simulink library "TB6612FNG"  (R2023b)
settings: Solver=VariableStepAuto  StartTime=0.0  StopTime=10.0  RelTol=1e-3
libraries: arduinolib x5
settings Model: Creator=user  LastModifiedBy=user

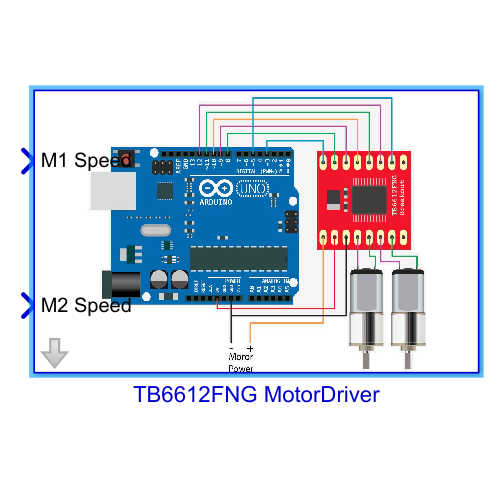
[thumbnail: Simulink's stored preview of the top-level diagram]
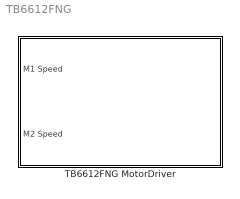
== system TB6612FNG ==
  TB6612FNG MotorDriver : Subsystem  mask{SetBYPin=8, InputAPin=7, EnablePin1=5, InputBPin=12, EnablePin2=6}
      mask TypeOptions SetBYPin: Digital Output2/pinNumber
      mask TypeOptions InputAPin: Digital Output/pinNumber
      mask TypeOptions EnablePin1: PWMSelection/pinNumber
      mask TypeOptions InputBPin: Digital Output1/pinNumber
      mask TypeOptions EnablePin2: PWMSelection1/pinNumber
      mask DialogControl DescGroupVar Prompt: TB6612FNG
      mask DialogControl DescTextVar Prompt: arduino：TB6612FNG Motor Driver
      mask Display: image('TB6612FNG.jpg');

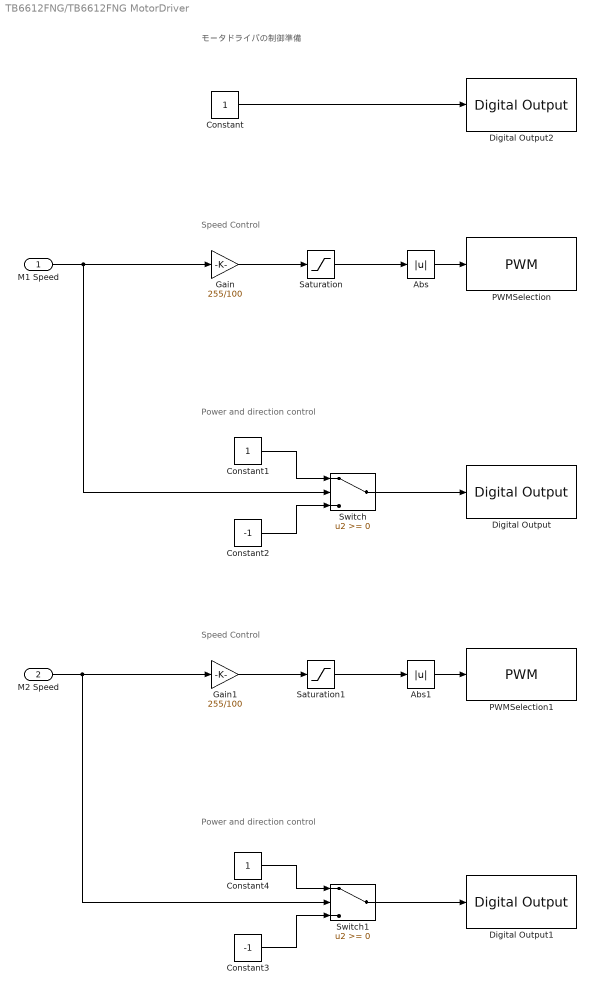
== system TB6612FNG/TB6612FNG MotorDriver ==
  note: Speed Control
  note: Power and direction control
  note: モータドライバの制御準備
  note: Power and direction control
  note: Speed Control
  M1 Speed : Inport
  M2 Speed : Inport  Port=2
  Abs : Abs  SaturateOnIntegerOverflow=off
  Abs1 : Abs  SaturateOnIntegerOverflow=off
  Constant : Constant
  Constant1 : Constant
  Constant2 : Constant  Value=-1
  Constant3 : Constant  Value=-1
  Constant4 : Constant
  Digital Output : arduinolib/Digital Output  pinNumber=InputAPin  Direction=output  blockPlatform=arduino
      settings: LibrarySourceBlock=arduinolib/L293D DC Motor/Digital Output
  Digital Output1 : arduinolib/Digital Output  pinNumber=InputBPin  Direction=output  blockPlatform=arduino
      settings: LibrarySourceBlock=arduinolib/L293D DC Motor/Digital Output
  Digital Output2 : arduinolib/Digital Output  pinNumber=SetBYPin  Direction=output  blockPlatform=arduino
  Gain : Gain  Gain=255/100
  Gain1 : Gain  Gain=255/100
  PWMSelection : arduinolib/PWM  pinNumber=EnablePin1  frequencyType=Default  desiredFrequency=490.2  achievableFrequency=490.2
      settings: LibrarySourceBlock=arduinolib/L293D DC Motor/PWMSelection
  PWMSelection1 : arduinolib/PWM  pinNumber=EnablePin2  frequencyType=Default  desiredFrequency=490.2  achievableFrequency=490.2
      settings: LibrarySourceBlock=arduinolib/L293D DC Motor/PWMSelection
  Saturation : Saturate  UpperLimit=255  LowerLimit=-255
  Saturation1 : Saturate  UpperLimit=255  LowerLimit=-255
  Switch : Switch  SaturateOnIntegerOverflow=off  InputSameDT=off
  Switch1 : Switch  SaturateOnIntegerOverflow=off  InputSameDT=off
  wires:
  Saturation/1 -> Abs/1
  M1 Speed/1 -> Switch/2, Gain/1
  Constant/1 -> Digital Output2/1
  Gain/1 -> Saturation/1
  Abs/1 -> PWMSelection/1
  Abs1/1 -> PWMSelection1/1
  Gain1/1 -> Saturation1/1
  Saturation1/1 -> Abs1/1
  Switch/1 -> Digital Output/1
  Switch1/1 -> Digital Output1/1
  Constant1/1 -> Switch/1
  Constant2/1 -> Switch/3
  Constant3/1 -> Switch1/3
  Constant4/1 -> Switch1/1
  M2 Speed/1 -> Gain1/1, Switch1/2
